simulink model "OperationalSpaceGravityCompensation"  (R2020a)
settings: Solver=VariableStepAuto  StartTime=0.0  StopTime=1.0  RelTol=1e-3
values from neighbouring files (symbols this model uses):
  g = 9.81    [params.m]
  KD = diag([  35   45   15    1     0   0])    [params.m]
  KP = diag([ 250  350  100   50     1   1])    [params.m]
libraries: vrlib x1
settings Model: Creator=Sebastiano  LastModifiedBy=Sebastiano

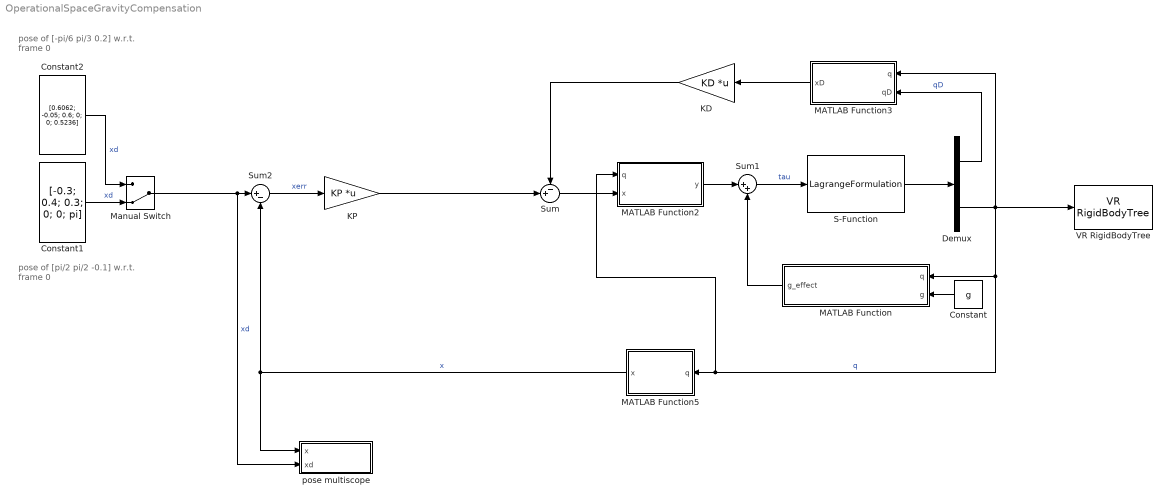
== system OperationalSpaceGravityCompensation ==
  note: pose of [pi/2 pi/2 -0.1]
      | w.r.t. frame 0
  note: pose of [-pi/6 pi/3 0.2]
      | w.r.t. frame 0
  Constant : Constant  Value=g
  Constant1 : Constant  Value=[-0.3; 0.4; 0.3; 0; 0; pi]  VectorParams1D=off
  Constant2 : Constant  Value=[0.6062; -0.05; 0.6; 0; 0; 0.5236]  VectorParams1D=off
  Demux : Demux  Outputs=[3, 3]
  KD : Gain  Gain=KD  Multiplication=Matrix(K*u) (u vector)
  KP : Gain  Gain=KP  Multiplication=Matrix(K*u) (u vector)
  MATLAB Function : MATLAB Function  TreatAsAtomicUnit=on
  MATLAB Function2 : MATLAB Function  TreatAsAtomicUnit=on
  MATLAB Function3 : MATLAB Function  TreatAsAtomicUnit=on
  MATLAB Function5 : MATLAB Function  TreatAsAtomicUnit=on
  Manual Switch : ManualSwitch  CurrentSetting=0
  S-Function : S-Function  FunctionName=LagrangeFormulation  Parameters=g  SFunctionDeploymentMode=off  EnableBusSupport=off
  Sum : Sum  Inputs=-+|
  Sum1 : Sum  Inputs=|++
  Sum2 : Sum  Inputs=|+-
  VR RigidBodyTree : vrlib/VR RigidBodyTree  RBT=robot  useRBT=on  Ts=-1  ForceViewerOpen=on
      settings: SourceProductBaseCode=SL
  pose multiscope : Subsystem
  wires:
  Demux/2 -> MATLAB Function3/1(q), VR RigidBodyTree/1, MATLAB Function2/1(q), MATLAB Function5/1(q), MATLAB Function/1(q)  "q"
  Demux/1 -> MATLAB Function3/2(qD)  "qD"
  KP/1 -> Sum/2
  Sum2/1 -> KP/1  "xerr"
  MATLAB Function/1(g_effect) -> Sum1/2
  Constant/1 -> MATLAB Function/2(g)
  S-Function/1 -> Demux/1
  Sum1/1 -> S-Function/1  "tau"
  Sum/1 -> MATLAB Function2/2(x)
  KD/1 -> Sum/1
  MATLAB Function2/1(y) -> Sum1/1
  MATLAB Function5/1(x) -> pose multiscope/1(x), Sum2/2  "x"
  MATLAB Function3/1(xD) -> KD/1
  Manual Switch/1 -> pose multiscope/2(xd), Sum2/1  "xd"
  Constant1/1 -> Manual Switch/2  "xd"
  Constant2/1 -> Manual Switch/1  "xd"

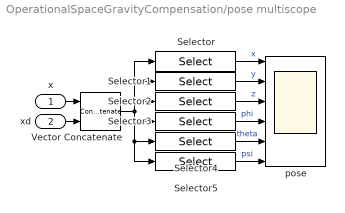
== system OperationalSpaceGravityCompensation/pose multiscope ==
  x : Inport
  xd : Inport  Port=2
  Selector : Selector  NumberOfDimensions=2  InputPortWidth=3  IndexOptions=Index vector (dialog),Select all  Indices=1,7  OutputSizes=6,6
  Selector1 : Selector  NumberOfDimensions=2  InputPortWidth=3  IndexOptions=Index vector (dialog),Select all  Indices=2,7  OutputSizes=6,6
  Selector2 : Selector  NumberOfDimensions=2  InputPortWidth=3  IndexOptions=Index vector (dialog),Select all  Indices=3,7  OutputSizes=6,6
  Selector3 : Selector  NumberOfDimensions=2  InputPortWidth=3  IndexOptions=Index vector (dialog),Select all  Indices=4,7  OutputSizes=6,6
  Selector4 : Selector  NumberOfDimensions=2  InputPortWidth=3  IndexOptions=Index vector (dialog),Select all  Indices=5,7  OutputSizes=6,6
  Selector5 : Selector  NumberOfDimensions=2  InputPortWidth=3  IndexOptions=Index vector (dialog),Select all  Indices=6,7  OutputSizes=6,6
  Vector Concatenate : Concatenate  Mode=Multidimensional array  ConcatenateDimension=2
  pose : Scope  NumInputPorts=6
  wires:
  x/1 -> Vector Concatenate/1
  xd/1 -> Vector Concatenate/2
  Selector1/1 -> pose/2  "y"
  Selector5/1 -> pose/6  "psi"
  Selector3/1 -> pose/4  "phi"
  Selector/1 -> pose/1  "x"
  Selector4/1 -> pose/5  "theta"
  Vector Concatenate/1 -> Selector/1, Selector1/1, Selector2/1, Selector5/1, Selector4/1, Selector3/1
  Selector2/1 -> pose/3  "z"

== matlab function OperationalSpaceGravityCompensation/MATLAB Function2 ==
  data: q input; y output; x input
function y = JAT(q, x)

y = AnalyticalJacobian(q)' * x;

== matlab function OperationalSpaceGravityCompensation/MATLAB Function3 ==
  data: q input; xD output; qD input
function xD = JA(q, qD)

xD = AnalyticalJacobian(q)*qD;

== matlab function OperationalSpaceGravityCompensation/MATLAB Function5 ==
  data: q input; x output
function x = K(q)

t1 = q(1);
t2 = q(2);
d3 = q(3);

% wrt frame 0
K = [[ cos(t1 + t2), -sin(t1 + t2), 0, (3*cos(t1 + t2))/10 + (2*cos(t1))/5]
     [ sin(t1 + t2),  cos(t1 + t2), 0, (3*sin(t1 + t2))/10 + (2*sin(t1))/5]
     [            0,             0, 1,                            d3 + 2/5]
     [            0,             0, 0,                                   1]];

pos = K(1:3, 4);
ori = rotm2eul(K(1:3,1:3), 'ZYZ')';

x = [pos; ori];

== matlab function OperationalSpaceGravityCompensation/MATLAB Function ==
  data: q input; g_effect output; g input
function g_effect = gravity(q, g)

g_effect = G_Lagrangian(q, g);
